simulink model "MultirotorSimulationController"  (R2015b)
settings: Solver=VariableStepAuto  StartTime=0.0  StopTime=Simulation.T_END  MaxStep=Simulation.TS_MAX  RelTol=1e-3
PreLoadFcn:
  | InitializeParameters;
undefined symbols (not defined in the file): Initial
libraries: Px4Library x13, QuaternionLibrary x7
settings Model: Creator=jban039  LastModifiedBy=jeremiebannwarth
settings DataIOCC: Decimation=10  LimitDataPoints=off
settings DebuggingCC: UnconnectedLineMsg=none
settings ModelReferenceCC: ModelReferenceMinAlgLoopOccurrences=on

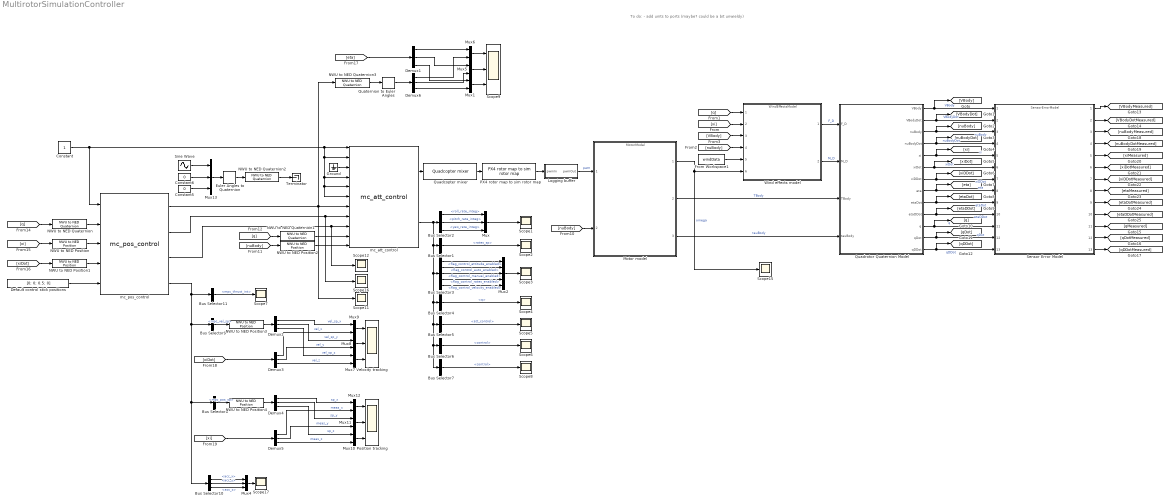
== system MultirotorSimulationController ==
  note: To do:
      |
      | - add units  to ports (maybe? could be a bit unwieldy)
  Bus Selector1 : BusSelector  OutputSignals=rates_sp
  Bus Selector10 : BusSelector  OutputSignals=mpc_local_pos_sp.acc_x,mpc_local_pos_sp.acc_y,mpc_local_pos_sp.acc_z
  Bus Selector11 : BusSelector  OutputSignals=mpc_thrust_int
  Bus Selector2 : BusSelector  OutputSignals=controller_status.roll_rate_integ,controller_status.pitch_rate_integ,controller_status.yaw_rate_integ
  Bus Selector3 : BusSelector  OutputSignals=v_control_mode.flag_control_attitude_enabled,v_control_mode.flag_control_auto_enabled,v_control_mode.flag_control_manual_enabled,v_control_mode.flag_control_rates_enabled,v_control_mode.flag_control_velocity_enabled
  Bus Selector4 : BusSelector  OutputSignals=ctrl_state.q
  Bus Selector5 : BusSelector  OutputSignals=att_control
  Bus Selector6 : BusSelector  OutputSignals=actuators.control
  Bus Selector7 : BusSelector  OutputSignals=actuators.control
  Bus Selector8 : BusSelector  OutputSignals=mpc_pos_sp
  Bus Selector9 : BusSelector  OutputSignals=mpc_vel_sp
  Constant : Constant
  Constant5 : Constant  Value=0
  Constant6 : Constant  Value=0
  Default control stick positions : Constant  Value=[0; 0; 0.5; 0]
  Demux{1..6} (6 alike) : Demux  Outputs=3
  Euler Angles to Quaternion : QuaternionLibrary/Euler Angles to Quaternion
  From Workspace1 : FromWorkspace  VariableName=windData  SampleTime=0
  Ground : Ground
  Logging buffer : Subsystem
  Motor model : ModelReference  ModelNameDialog=MotorModel  SimulationMode=Normal  ModelReferenceVersion=1.136  CopyOfModelName=MotorModel
  Mux : Mux  Inputs=3
  Mux{1,5..12} (9 alike) : Mux  Inputs=2
  Mux13 : Mux  Inputs=3
  Mux2 : Mux  Inputs=5
  Mux4 : Mux  Inputs=3
  NWU to NED Position{,1..4} (5 alike) : Px4Library/NWU to NED Position
  NWU to NED Quaternion{,1..3} (4 alike) : Px4Library/NWU to NED Quaternion
  PX4 rotor map to sim rotor map : Px4Library/PX4 rotor map to sim rotor map  SystemSampleTime=-1
  Position tracking : Scope  NumInputPorts=3
  Quadcopter mixer : Px4Library/Quadcopter mixer  MC_SAMPLING_PERIOD=0.002
  Quadrotor Quaternion Model : Subsystem
  Quaternion to Euler Angles : QuaternionLibrary/Quaternion to Euler Angles
  Scope{1..8,11..12,15..17} (13 alike) : Scope
  Scope9 : Scope  NumInputPorts=3
  Sensor Error Model : ModelReference  ModelNameDialog=SensorErrorModel  SimulationMode=Normal  ModelReferenceVersion=1.5  CopyOfModelName=SensorErrorModel
  Sine Wave : Sin  Amplitude=10*pi/180  SampleTime=0
  Terminator : Terminator
  Velocity tracking : Scope  NumInputPorts=3
  Wind effects model : ModelReference  ModelNameDialog=WindEffectsModel  SimulationMode=Normal  ModelReferenceVersion=1.67  CopyOfModelName=WindEffectsModel
  mc_att_control : Px4Library/mc_att_control  MC_SAMPLING_PERIOD=0.002  MC_ROLL_TC=0.2  MC_PITCH_TC=0.2  MC_ROLL_P=6.5  MC_ROLLRATE_P=0.15  MC_ROLLRATE_I=0.05  MC_ROLLRATE_D=0.003  MC_ROLLRATE_FF=0.0  MC_PITCH_P=6.5  MC_PITCHRATE_P=0.15  MC_PITCHRATE_I=0.05  MC_PITCHRATE_D=0.003  MC_PITCHRATE_FF=0.0  MC_YAW_P=2.8  MC_YAWRATE_P=0.2  MC_YAWRATE_I=0.1  MC_YAWRATE_D=0.0  MC_YAWRATE_FF=0.0  MC_YAW_FF=0.5  MC_ROLLRATE_MAX=220.0  MC_PITCHRATE_MAX=220.0  MC_YAWRATE_MAX=200.0  MC_YAWRAUTO_MAX=45.0  MC_ACRO_R_MAX=360.0  MC_ACRO_P_MAX=360.0  MC_ACRO_Y_MAX=360.0  MC_RATT_TH=1.0  MC_TPA_BREAK=1.0  MC_TPA_SLOP=1.0  VT_OPT_RECOV_EN=0.0  VT_WV_YAWR_SCL=0.15  MC_RR_INT_LIM=0.30  MC_PR_INT_LIM=0.30  MC_TPA_BREAK_P=1.0  MC_TPA_BREAK_I=1.0  MC_TPA_BREAK_D=1.0  MC_TPA_RATE_P=0.0  MC_TPA_RATE_I=0.0  MC_TPA_RATE_D=0.0  VT_TYPE=2  MC_BAT_SCALE_EN=0  MC_YR_INT_LIM=0.30
  mc_pos_control : Px4Library/mc_pos_control  THROTTLE_HOVER=Uav.THROTTLE_HOVER  MPC_SAMPLING_PERIOD=0.02  MPC_THR_MIN=0.120  MPC_THR_HOVER=0.500  MPC_ALTCTL_DZ=0.100  MPC_ALTCTL_DY=0.0  MPC_THR_MAX=0.900  MPC_MANTHR_MIN=0.080  MPC_MANTHR_MAX=0.900  MPC_Z_P=1.000  MPC_Z_VEL_P=0.200  MPC_Z_VEL_I=0.020  MPC_Z_VEL_D=0.0  MPC_Z_VEL_MAX_UP=3.0  MPC_Z_VEL_MAX=1.000  MPC_Z_VEL_MAX_DN=1.000  MPC_Z_FF=0.500  MPC_XY_P=0.950  MPC_XY_VEL_P=0.090  MPC_XY_VEL_I=0.020  MPC_XY_VEL_D=0.010  MPC_XY_CRUISE=5.0  MPC_XY_VEL_MAX=8.0  MPC_XY_FF=0.500  MPC_TILTMAX_AIR=45.0  MPC_TILTMAX_LND=12.0  MPC_LAND_SPEED=0.500  MPC_TKO_SPEED=1.500  MPC_MAN_R_MAX=35.0  MPC_MAN_P_MAX=35.0  MPC_MAN_Y_MAX=200.0  MPC_HOLD_XY_DZ=0.100  MPC_HOLD_MAX_XY=0.800  MPC_HOLD_MAX_Z=0.600  MPC_VELD_LP=5.0  MPC_ACC_HOR_MAX=5.0  MPC_ALT_MODE=0.0  MC_YAWRATE_MAX=200.0  MC_YAW_P=2.800  VT_OPT_RECOV_EN=0.0
  wires:
  Motor model/1 -> Wind effects model/6, Scope15/1  "omega"
  Motor model/2 -> Quadrotor Quaternion Model/3(TBody)  "TBody"
  Motor model/3 -> Quadrotor Quaternion Model/4(tauBody)  "tauBody"
  Wind effects model/2 -> Quadrotor Quaternion Model/2(M_D)  "M_D"
  Quadrotor Quaternion Model/1(VBody) -> Sensor Error Model/1, [VBody]  "VBody"
  Quadrotor Quaternion Model/2(VBodyDot) -> Sensor Error Model/2, [VBodyDot]  "VBodyDot"
  Quadrotor Quaternion Model/3(nuBody) -> [nuBody], Sensor Error Model/3  "nuBody"
  Quadrotor Quaternion Model/4(nuBodyDot) -> Sensor Error Model/4, [nuBodyDot]  "nuBodyDot"
  Quadrotor Quaternion Model/5(xi) -> Sensor Error Model/5, [xi]  "xi"
  Quadrotor Quaternion Model/6(xiDot) -> Sensor Error Model/6, [xiDot]  "xiDot"
  Quadrotor Quaternion Model/7(xiDDot) -> Sensor Error Model/7, [xiDDot]  "xiDDot"
  Quadrotor Quaternion Model/8(eta) -> Sensor Error Model/8, [eta]  "eta"
  Quadrotor Quaternion Model/9(etaDot) -> Sensor Error Model/9, [etaDot]  "etaDot"
  Quadrotor Quaternion Model/10(etaDDot) -> [etaDDot], Sensor Error Model/10  "etaDDot"
  [q] -> Wind effects model/1
  [xi] -> Wind effects model/2
  [nuBody] -> Wind effects model/4
  [VBody] -> Wind effects model/3
  [nuBody] -> Motor model/2
  Quadrotor Quaternion Model/11(q) -> Sensor Error Model/11, [q]  "q"
  Quadrotor Quaternion Model/12(qDot) -> [qDot], Sensor Error Model/12  "qDot"
  Quadrotor Quaternion Model/13(qDDot) -> Sensor Error Model/13, [qDDot]  "qDDot"
  Wind effects model/1 -> Quadrotor Quaternion Model/1(F_D)  "F_D"
  Sensor Error Model/1 -> [VBodyMeasured]
  Sensor Error Model/2 -> [VBodyDotMeasured]
  Sensor Error Model/3 -> [nuBodyMeasured]
  Sensor Error Model/4 -> [nuBodyDotMeasured]
  Sensor Error Model/5 -> [xiMeasured]
  Sensor Error Model/6 -> [xiDotMeasured]
  Sensor Error Model/7 -> [xiDDotMeasured]
  Sensor Error Model/8 -> [etaMeasured]
  Sensor Error Model/9 -> [etaDotMeasured]
  Sensor Error Model/10 -> [etaDDotMeasured]
  Sensor Error Model/11 -> [qMeasured]
  Sensor Error Model/12 -> [qDotMeasured]
  Sensor Error Model/13 -> [qDDotMeasured]
  Logging buffer/1(pwmOut) -> Motor model/1  "pwm"
  [nuBody] -> NWU to NED Position2/1
  Constant/1 -> mc_att_control/4, mc_att_control/5, mc_att_control/6, mc_att_control/2, mc_att_control/1, mc_pos_control/1
  Bus Selector2/1 -> Mux/1  "<roll_rate_integ>"
  Bus Selector2/2 -> Mux/2  "<pitch_rate_integ>"
  Bus Selector2/3 -> Mux/3  "<yaw_rate_integ>"
  Mux/1 -> Scope1/1
  mc_att_control/2 -> Bus Selector7/1, Bus Selector6/1, Bus Selector5/1, Bus Selector4/1, Bus Selector3/1, Bus Selector1/1, Bus Selector2/1
  Bus Selector1/1 -> Scope2/1  "<rates_sp>"
  Bus Selector3/1 -> Mux2/1  "<flag_control_attitude_enabled>"
  Bus Selector3/2 -> Mux2/2  "<flag_control_auto_enabled>"
  Bus Selector3/3 -> Mux2/3  "<flag_control_manual_enabled>"
  Bus Selector3/4 -> Mux2/4  "<flag_control_rates_enabled>"
  Bus Selector3/5 -> Mux2/5  "<flag_control_velocity_enabled>"
  Mux2/1 -> Scope3/1
  Bus Selector4/1 -> Scope4/1  "<q>"
  Bus Selector5/1 -> Scope5/1  "<att_control>"
  Bus Selector6/1 -> Scope6/1  "<control>"
  Bus Selector7/1 -> Scope8/1  "<control>"
  mc_pos_control/1 -> NWU to NED Quaternion3/1, Scope11/1, mc_att_control/7
  mc_pos_control/4 -> Bus Selector11/1, Bus Selector10/1, Bus Selector8/1, Bus Selector9/1
  [q] -> NWU to NED Quaternion/1
  [xiDot] -> NWU to NED Position1/1
  Default control stick positions/1 -> mc_pos_control/5
  [q] -> NWU to NED Quaternion1/1
  NWU to NED Quaternion1/1 -> mc_att_control/10
  NWU to NED Position2/1 -> mc_att_control/11
  NWU to NED Quaternion/1 -> mc_pos_control/2
  mc_pos_control/3 -> mc_att_control/9, Scope12/1
  mc_pos_control/2 -> Scope16/1, mc_att_control/8
  Mux1/1 -> Scope9/3
  Bus Selector9/1 -> NWU to NED Position3/1  "<mpc_vel_sp>"
  NWU to NED Position1/1 -> mc_pos_control/4
  NWU to NED Position/1 -> mc_pos_control/3
  [xi] -> NWU to NED Position/1
  Bus Selector10/1 -> Mux4/1  "<acc_x>"
  Bus Selector10/2 -> Mux4/2  "<acc_y>"
  Bus Selector10/3 -> Mux4/3  "<acc_z>"
  Mux4/1 -> Scope17/1
  Mux5/1 -> Scope9/2
  Mux6/1 -> Scope9/1
  [eta] -> Demux1/1
  Demux1/1 -> Mux6/1
  Demux1/2 -> Mux5/1
  Mux7/1 -> Velocity tracking/3
  Mux8/1 -> Velocity tracking/2
  Mux9/1 -> Velocity tracking/1
  [xiDot] -> Demux3/1
  Demux2/1 -> Mux9/1  "vel_sp_x"
  Demux3/1 -> Mux9/2  "vel_x"
  Demux2/2 -> Mux8/1  "vel_sp_y"
  Demux3/2 -> Mux8/2  "vel_y"
  Demux2/3 -> Mux7/1  "vel_sp_z"
  Demux3/3 -> Mux7/2  "vel_z"
  Mux10/1 -> Position tracking/3
  Mux11/1 -> Position tracking/2
  Mux12/1 -> Position tracking/1
  [xi] -> Demux5/1
  Demux4/1 -> Mux12/1  "sp_x"
  Demux5/1 -> Mux12/2  "meas_x"
  Demux4/2 -> Mux11/1  "sp_y"
  Demux5/2 -> Mux11/2  "meas_y"
  Demux4/3 -> Mux10/1  "sp_z"
  Demux5/3 -> Mux10/2  "meas_z"
  Mux13/1 -> Euler Angles to Quaternion/1
  Constant5/1 -> Mux13/3
  Constant6/1 -> Mux13/2
  Sine Wave/1 -> Mux13/1
  Quaternion to Euler Angles/1 -> Demux6/1
  Demux6/1 -> Mux6/2
  Demux6/2 -> Mux5/2
  Demux6/3 -> Mux1/2
  Demux1/3 -> Mux1/1
  Euler Angles to Quaternion/1 -> NWU to NED Quaternion2/1
  NWU to NED Quaternion3/1 -> Quaternion to Euler Angles/1
  Ground/1 -> mc_att_control/3
  mc_att_control/1 -> Quadcopter mixer/1
  Quadcopter mixer/1 -> PX4 rotor map to sim rotor map/1
  PX4 rotor map to sim rotor map/1 -> Logging buffer/1(pwmIn)
  Bus Selector8/1 -> NWU to NED Position4/1  "<mpc_pos_sp>"
  NWU to NED Quaternion2/1 -> Terminator/1
  Bus Selector11/1 -> Scope7/1  "<mpc_thrust_int>"
  NWU to NED Position3/1 -> Demux2/1
  NWU to NED Position4/1 -> Demux4/1
  From Workspace1/1 -> Wind effects model/5

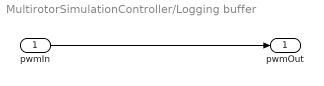
== system MultirotorSimulationController/Logging buffer ==
  pwmIn : Inport
  pwmOut : Outport
  wires:
  pwmIn/1 -> pwmOut/1

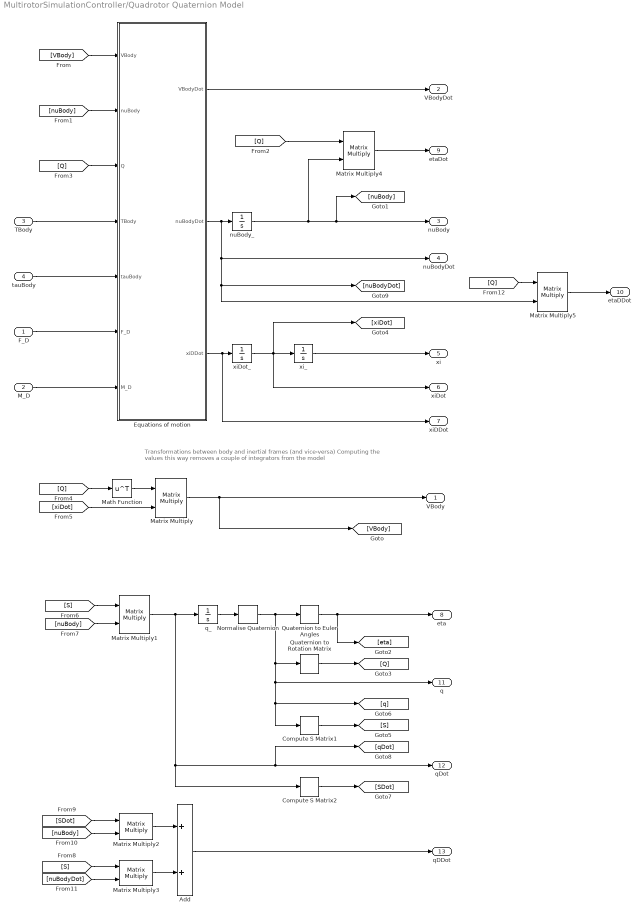
== system MultirotorSimulationController/Quadrotor Quaternion Model ==
  note: Transformations between body and inertial frames (and vice-versa)
      | Computing the values this way removes a couple of integrators from the model
  F_D : Inport
  M_D : Inport  Port=2
  TBody : Inport  Port=3
  tauBody : Inport  Port=4
  Add : Sum
  Compute S Matrix1 : QuaternionLibrary/Compute S Matrix
  Compute S Matrix2 : QuaternionLibrary/Compute S Matrix
  Equations of motion : MATLAB Function  TreatAsAtomicUnit=on
  Math Function : Math  Operator=transpose  SaturateOnIntegerOverflow=on
  Matrix Multiply{,1..5} (6 alike) : Product  Multiplication=Matrix(*)
  Normalise Quaternion : QuaternionLibrary/Normalise Quaternion
  Quaternion to Euler Angles : QuaternionLibrary/Quaternion to Euler Angles
  Quaternion to Rotation Matrix : QuaternionLibrary/Quaternion to Rotation Matrix
  nuBody_ : Integrator  InitialCondition=Initial.NU_BODY
  q_ : Integrator  InitialCondition=Initial.Q
  xiDot_ : Integrator  InitialCondition=Initial.XI_DOT
  xi_ : Integrator  InitialCondition=Initial.XI
  VBody : Outport
  VBodyDot : Outport  Port=2
  nuBody : Outport  Port=3
  nuBodyDot : Outport  Port=4
  xi : Outport  Port=5
  xiDot : Outport  Port=6
  xiDDot : Outport  Port=7
  eta : Outport  Port=8
  etaDot : Outport  Port=9
  etaDDot : Outport  Port=10
  q : Outport  Port=11
  qDot : Outport  Port=12
  qDDot : Outport  Port=13
  wires:
  Equations of motion/1(VBodyDot) -> VBodyDot/1
  xiDot_/1 -> xi_/1, [xiDot], xiDot/1
  xi_/1 -> xi/1
  [nuBody] -> Equations of motion/2(nuBody)
  [VBody] -> Equations of motion/1(VBody)
  tauBody/1 -> Equations of motion/5(tauBody)
  TBody/1 -> Equations of motion/4(TBody)
  Equations of motion/3(xiDDot) -> xiDot_/1, xiDDot/1
  F_D/1 -> Equations of motion/6(F_D)
  Matrix Multiply/1 -> VBody/1, [VBody]
  M_D/1 -> Equations of motion/7(M_D)
  nuBody_/1 -> Matrix Multiply4/2, [nuBody], nuBody/1
  Equations of motion/2(nuBodyDot) -> nuBody_/1, nuBodyDot/1, Matrix Multiply5/2, [nuBodyDot]
  q_/1 -> Normalise Quaternion/1
  Quaternion to Euler Angles/1 -> eta/1, [eta]
  Matrix Multiply4/1 -> etaDot/1
  Quaternion to Rotation Matrix/1 -> [Q]
  [Q] -> Equations of motion/3(Q)
  [Q] -> Math Function/1
  [xiDot] -> Matrix Multiply/2
  Math Function/1 -> Matrix Multiply/1
  [S] -> Matrix Multiply1/1
  [nuBody] -> Matrix Multiply1/2
  Compute S Matrix2/1 -> [SDot]
  [S] -> Matrix Multiply3/1
  Matrix Multiply1/1 -> qDot/1, [qDot], Compute S Matrix2/1, q_/1
  [SDot] -> Matrix Multiply2/1
  [nuBody] -> Matrix Multiply2/2
  [nuBodyDot] -> Matrix Multiply3/2
  Matrix Multiply2/1 -> Add/1
  Matrix Multiply3/1 -> Add/2
  Normalise Quaternion/1 -> Quaternion to Euler Angles/1, q/1, Compute S Matrix1/1, [q], Quaternion to Rotation Matrix/1
  Compute S Matrix1/1 -> [S]
  [Q] -> Matrix Multiply4/1
  Add/1 -> qDDot/1
  [Q] -> Matrix Multiply5/1
  Matrix Multiply5/1 -> etaDDot/1

== matlab function MultirotorSimulationController/Quadrotor Quaternion Model/Equations of motion ==
  data: VBody input; VBodyDot output; nuBody input; Q input; TBody input size=3; tauBody input size=3; F_D input size=3; M_D input size=3; nuBodyDot output; Uav parameter; xiDDot output
function [VBodyDot, nuBodyDot, xiDDot] = QuadrotorQuaternionModel(...
    VBody, nuBody, Q, TBody, tauBody, F_D, M_D, Uav)
%#codegen

%% Rotation matrices

%% Moments and Forces
% Body frame accelerations
VBodyDot  = (1/Uav.M) * (Q'*Uav.G + TBody - cross(nuBody, Uav.M*VBody) - F_D);
nuBodyDot = Uav.I \ (tauBody - cross(nuBody, Uav.I*nuBody) - M_D);

% Inertial frame accelerations
xiDDot = (1/Uav.M)*(Uav.G + Q*(TBody - F_D));
% etaDDot = WInvertDot*nuBody + WInvert*nuBodyDot;

% Check centripetal force in inertial frame
% F_C = R*cross(nuBody,m*VBody);
end
